simulink model "Centralized_Cont"  (R2018a)
settings: Solver=VariableStepAuto  StartTime=0.0  StopTime=5  RelTol=1e-3
values from neighbouring files (symbols this model uses):
  Kd_Cent = zeros(7,7)    [ControlSetup.m]
  Kp_Cent = zeros(7,7)    [ControlSetup.m]
libraries: dspinverses x1
(part 1 of 4)
settings Model: Creator=Pedro Ramalho  LastModifiedBy=Pedro Ramalho
settings DataIOCC: ReturnWorkspaceOutputs=on  ReturnWorkspaceOutputsName=Centralized

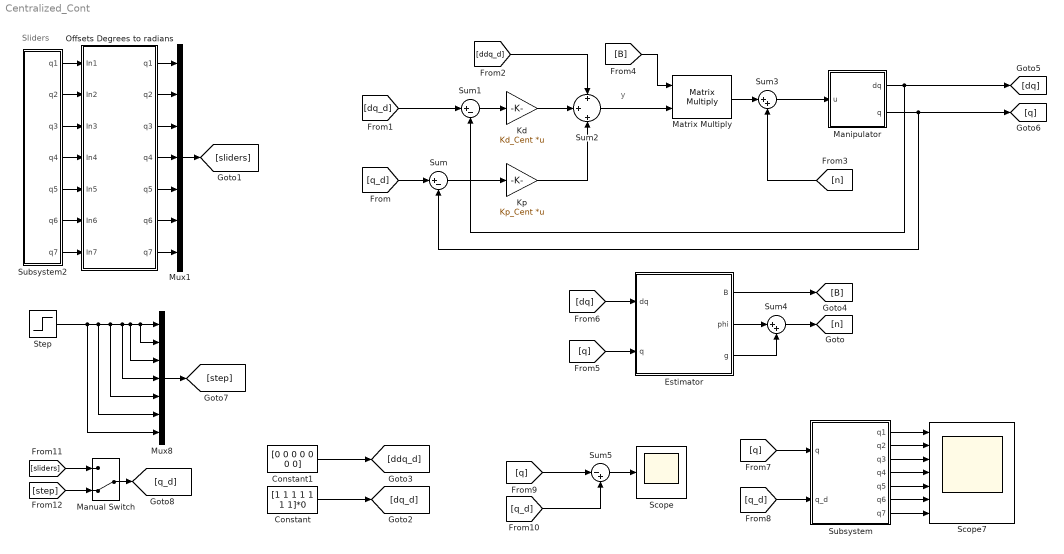
== system Centralized_Cont ==
  note: y
  note: Sliders
  Constant : Constant  Value=[1 1 1 1 1 1 1]*0  OutDataTypeStr=int16  SampleTime=-1
  Constant1 : Constant  Value=[0 0 0 0 0 0 0]  OutDataTypeStr=int16  SampleTime=-1
  Estimator : Subsystem
  Kd : Gain  Gain=Kd_Cent  Multiplication=Matrix(K*u)
  Kp : Gain  Gain=Kp_Cent  Multiplication=Matrix(K*u)
  Manipulator : Subsystem
  Manual Switch : ManualSwitch  CurrentSetting=0
  Matrix Multiply : Product  Multiplication=Matrix(*)
  Mux1 : Mux  Inputs=7
  Mux8 : Mux  Inputs=7
  Offsets Degrees to radians : Subsystem
  Scope : Scope
  Scope7 : Scope  NumInputPorts=7
  Step : Step  SampleTime=0
  Subsystem : Subsystem
  Subsystem2 : Subsystem  mask{q1=1.0, q2=82.800, q3=180.0, q4=-180.0, q5=-180.0, q6=-180.0, q7=180.0}
  Sum : Sum  Inputs=|+-
  Sum1 : Sum  Inputs=|+-
  Sum2 : Sum  Inputs=+|+|+
  Sum3 : Sum  Inputs=|++
  Sum4 : Sum  Inputs=|++
  Sum5 : Sum  Inputs=|-+
  wires:
  Subsystem2/5(q5) -> Offsets Degrees to radians/5(In5)
  Offsets Degrees to radians/1(q1) -> Mux1/1
  Subsystem2/2(q2) -> Offsets Degrees to radians/2(In2)
  Offsets Degrees to radians/2(q2) -> Mux1/2
  Subsystem2/3(q3) -> Offsets Degrees to radians/3(In3)
  Subsystem2/4(q4) -> Offsets Degrees to radians/4(In4)
  Subsystem2/1(q1) -> Offsets Degrees to radians/1(In1)
  Offsets Degrees to radians/7(q7) -> Mux1/7
  Offsets Degrees to radians/6(q6) -> Mux1/6
  Offsets Degrees to radians/3(q3) -> Mux1/3
  Subsystem2/7(q7) -> Offsets Degrees to radians/7(In7)
  Mux1/1 -> [sliders]
  Offsets Degrees to radians/5(q5) -> Mux1/5
  Subsystem2/6(q6) -> Offsets Degrees to radians/6(In6)
  Offsets Degrees to radians/4(q4) -> Mux1/4
  Constant/1 -> [dq_d]
  Constant1/1 -> [ddq_d]
  [q_d] -> Sum/1
  [dq_d] -> Sum1/1
  Sum1/1 -> Kd/1
  Kd/1 -> Sum2/2
  Kp/1 -> Sum2/3
  Estimator/2(phi) -> Sum4/1
  Estimator/3(g) -> Sum4/2
  Sum4/1 -> [n]
  Matrix Multiply/1 -> Sum3/1
  [n] -> Sum3/2
  Estimator/1(B) -> [B]
  [B] -> Matrix Multiply/1
  Sum3/1 -> Manipulator/1(u)
  [q] -> Estimator/2(q)
  [dq] -> Estimator/1(dq)
  [q] -> Sum5/1
  [q_d] -> Sum5/2
  Sum5/1 -> Scope/1
  Step/1 -> Mux8/7, Mux8/6, Mux8/5, Mux8/4, Mux8/1, Mux8/2, Mux8/3
  Mux8/1 -> [step]
  Sum/1 -> Kp/1
  Sum2/1 -> Matrix Multiply/2
  [ddq_d] -> Sum2/1
  [q] -> Subsystem/1(q)
  [q_d] -> Subsystem/2(q_d)
  Subsystem/1(q1) -> Scope7/1
  Subsystem/2(q2) -> Scope7/2
  Subsystem/3(q3) -> Scope7/3
  Subsystem/4(q4) -> Scope7/4
  Subsystem/5(q5) -> Scope7/5
  Subsystem/6(q6) -> Scope7/6
  Subsystem/7(q7) -> Scope7/7
  Manipulator/2(q) -> [q], Sum/2
  Manipulator/1(dq) -> [dq], Sum1/2
  [sliders] -> Manual Switch/1
  [step] -> Manual Switch/2
  Manual Switch/1 -> [q_d]

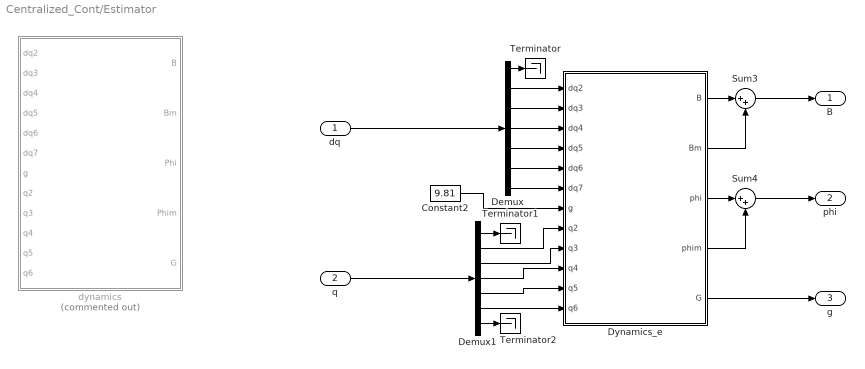
== system Centralized_Cont/Estimator ==
  dq : Inport
  q : Inport  Port=2
  Constant2 : Constant  Value=9.81  SampleTime=-1
  Demux : Demux  Outputs=7
  Demux1 : Demux  Outputs=7
  Dynamics_e : MATLAB Function  TreatAsAtomicUnit=on
  Sum3 : Sum  Inputs=|++
  Sum4 : Sum  Inputs=|++
  Terminator : Terminator
  Terminator1 : Terminator
  Terminator2 : Terminator
  dynamics : MATLAB Function  Commented=on  TreatAsAtomicUnit=on
  B : Outport
  phi : Outport  Port=2
  g : Outport  Port=3
  wires:
  Demux1/7 -> Terminator2/1
  Demux/1 -> Terminator/1
  Demux1/1 -> Terminator1/1
  Demux/2 -> Dynamics_e/1(dq2)
  Demux/3 -> Dynamics_e/2(dq3)
  Demux/4 -> Dynamics_e/3(dq4)
  Demux/5 -> Dynamics_e/4(dq5)
  Demux/6 -> Dynamics_e/5(dq6)
  Demux/7 -> Dynamics_e/6(dq7)
  Dynamics_e/1(B) -> Sum3/1
  Dynamics_e/3(phi) -> Sum4/1
  Constant2/1 -> Dynamics_e/7(g)
  Demux1/2 -> Dynamics_e/8(q2)
  Demux1/3 -> Dynamics_e/9(q3)
  Demux1/4 -> Dynamics_e/10(q4)
  Demux1/5 -> Dynamics_e/11(q5)
  Demux1/6 -> Dynamics_e/12(q6)
  Dynamics_e/2(Bm) -> Sum3/2
  Dynamics_e/4(phim) -> Sum4/2
  dq/1 -> Demux/1
  q/1 -> Demux1/1
  Sum3/1 -> B/1
  Sum4/1 -> phi/1
  Dynamics_e/5(G) -> g/1

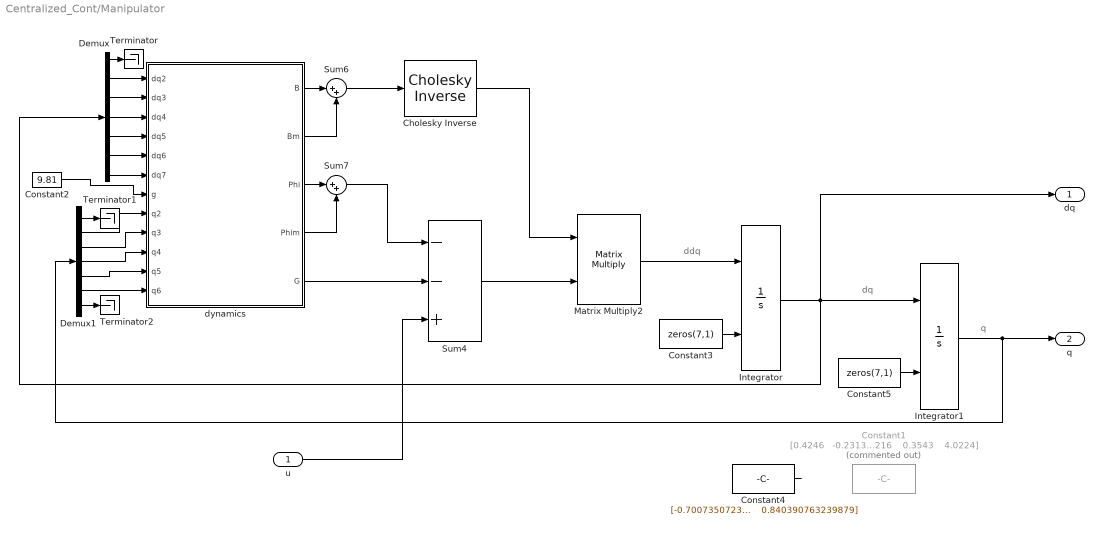
== system Centralized_Cont/Manipulator ==
  note: ddq
  note: dq
  note: q
  u : Inport
  Cholesky Inverse : dspinverses/Cholesky Inverse  errmode=Warning
      settings: SourceProductName=DSP System Toolbox  SourceProductBaseCode=DS
  Constant1 : Constant  Commented=on  Value="[0.4246   -0.2313   -1.6935   -0.1482    0.7216    0.3543    4.0224]"  SampleTime=-1
  Constant2 : Constant  Value=9.81  SampleTime=-1
  Constant3 : Constant  Value=zeros(7,1)  SampleTime=-1
  Constant4 : Constant  Value="[-0.700735072364346    0.260226322165590    -1.41409718169695    0.123044715609812    0.767247092108692    -0.379724450954367    0.840390763239879]"  SampleTime=-1
  Constant5 : Constant  Value=zeros(7,1)  SampleTime=-1
  Demux : Demux  Outputs=7
  Demux1 : Demux  Outputs=7
  Integrator : Integrator  InitialConditionSource=external
  Integrator1 : Integrator  InitialConditionSource=external
  Matrix Multiply2 : Product  Multiplication=Matrix(*)
  Sum4 : Sum  Inputs=--+
  Sum6 : Sum  Inputs=|++
  Sum7 : Sum  Inputs=|++
  Terminator : Terminator
  Terminator1 : Terminator
  Terminator2 : Terminator
  dynamics : MATLAB Function  TreatAsAtomicUnit=on
  dq : Outport
  q : Outport  Port=2
  wires:
  Demux/1 -> Terminator/1
  Cholesky Inverse/1 -> Matrix Multiply2/1
  Demux1/5 -> dynamics/11(q5)
  Sum4/1 -> Matrix Multiply2/2
  Sum7/1 -> Sum4/1
  Demux1/1 -> Terminator1/1
  Constant3/1 -> Integrator/2
  dynamics/5(G) -> Sum4/2
  Demux/2 -> dynamics/1(dq2)
  Demux1/7 -> Terminator2/1
  Matrix Multiply2/1 -> Integrator/1
  Demux1/4 -> dynamics/10(q4)
  Integrator/1 -> dq/1, Integrator1/1, Demux/1
  Demux1/2 -> dynamics/8(q2)
  Constant2/1 -> dynamics/7(g)
  Sum6/1 -> Cholesky Inverse/1
  Demux/3 -> dynamics/2(dq3)
  Constant4/1 -> ?
  dynamics/4(Phim) -> Sum7/2
  dynamics/3(Phi) -> Sum7/1
  Demux1/6 -> dynamics/12(q6)
  Demux/7 -> dynamics/6(dq7)
  dynamics/2(Bm) -> Sum6/2
  Demux/5 -> dynamics/4(dq5)
  dynamics/1(B) -> Sum6/1
  Demux1/3 -> dynamics/9(q3)
  Demux/4 -> dynamics/3(dq4)
  Demux/6 -> dynamics/5(dq6)
  Integrator1/1 -> q/1, Demux1/1
  u/1 -> Sum4/3
  Constant5/1 -> Integrator1/2

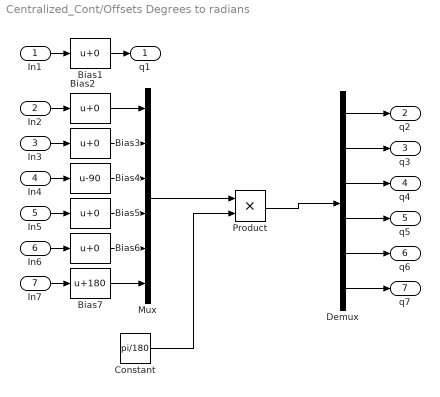
== system Centralized_Cont/Offsets Degrees to radians ==
  In1 : Inport
  In2 : Inport  Port=2
  In3 : Inport  Port=3
  In4 : Inport  Port=4
  In5 : Inport  Port=5
  In6 : Inport  Port=6
  In7 : Inport  Port=7
  Bias{1..3,5..6} (5 alike) : Bias
  Bias4 : Bias  Bias=-90
  Bias7 : Bias  Bias=180
  Constant : Constant  Value=pi/180
  Demux : Demux  Outputs=6
  Mux : Mux  Inputs=6
  Product : Product
  q1 : Outport
  q2 : Outport  Port=2
  q3 : Outport  Port=3
  q4 : Outport  Port=4
  q5 : Outport  Port=5
  q6 : Outport  Port=6
  q7 : Outport  Port=7
  wires:
  In6/1 -> Bias6/1
  In5/1 -> Bias5/1
  In3/1 -> Bias3/1
  In1/1 -> Bias1/1
  Bias1/1 -> q1/1
  In7/1 -> Bias7/1
  In4/1 -> Bias4/1
  In2/1 -> Bias2/1
  Bias7/1 -> Mux/6
  Bias2/1 -> Mux/1
  Bias3/1 -> Mux/2
  Bias4/1 -> Mux/3
  Bias5/1 -> Mux/4
  Bias6/1 -> Mux/5
  Mux/1 -> Product/1
  Constant/1 -> Product/2
  Demux/1 -> q2/1
  Demux/2 -> q3/1
  Demux/3 -> q4/1
  Demux/4 -> q5/1
  Demux/5 -> q6/1
  Demux/6 -> q7/1
  Product/1 -> Demux/1

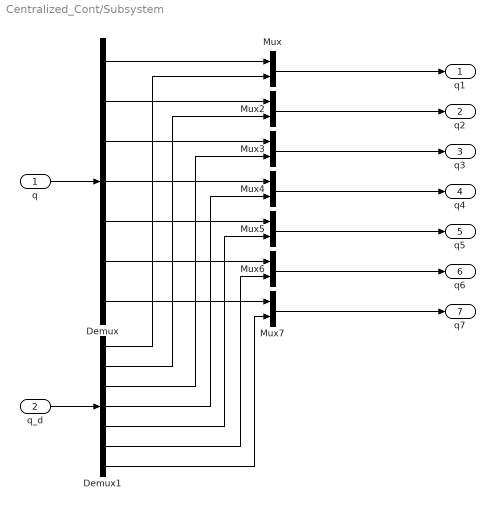
== system Centralized_Cont/Subsystem ==
  q : Inport
  q_d : Inport  Port=2
  Demux : Demux  Outputs=7
  Demux1 : Demux  Outputs=7
  Mux{,2..7} (7 alike) : Mux  Inputs=2
  q1 : Outport
  q2 : Outport  Port=2
  q3 : Outport  Port=3
  q4 : Outport  Port=4
  q5 : Outport  Port=5
  q6 : Outport  Port=6
  q7 : Outport  Port=7
  wires:
  Demux/3 -> Mux3/1
  Demux/7 -> Mux7/1
  Demux1/6 -> Mux6/2
  Demux1/1 -> Mux/2
  Demux/4 -> Mux4/1
  Demux1/4 -> Mux4/2
  Demux/1 -> Mux/1
  Demux1/5 -> Mux5/2
  Mux4/1 -> q4/1
  Demux1/3 -> Mux3/2
  Demux/2 -> Mux2/1
  Demux1/7 -> Mux7/2
  Demux1/2 -> Mux2/2
  Demux/5 -> Mux5/1
  Demux/6 -> Mux6/1
  Mux6/1 -> q6/1
  q/1 -> Demux/1
  Mux/1 -> q1/1
  Mux3/1 -> q3/1
  Mux2/1 -> q2/1
  Mux5/1 -> q5/1
  Mux7/1 -> q7/1
  q_d/1 -> Demux1/1

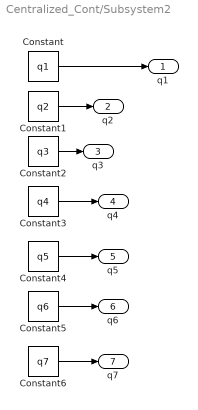
== system Centralized_Cont/Subsystem2 ==
  Constant : Constant  Value=q1
  Constant1 : Constant  Value=q2
  Constant2 : Constant  Value=q3
  Constant3 : Constant  Value=q4
  Constant4 : Constant  Value=q5
  Constant5 : Constant  Value=q6
  Constant6 : Constant  Value=q7
  q1 : Outport
  q2 : Outport  Port=2
  q3 : Outport  Port=3
  q4 : Outport  Port=4
  q5 : Outport  Port=5
  q6 : Outport  Port=6
  q7 : Outport  Port=7
  wires:
  Constant/1 -> q1/1
  Constant2/1 -> q3/1
  Constant1/1 -> q2/1
  Constant3/1 -> q4/1
  Constant4/1 -> q5/1
  Constant5/1 -> q6/1
  Constant6/1 -> q7/1
